simulink model "ODE1_zad1"  (Simulink 6.3)
settings: Solver=ode45  StartTime=0.0  StopTime=1  RelTol=1e-3
settings Model: LastModifiedBy=Ms1

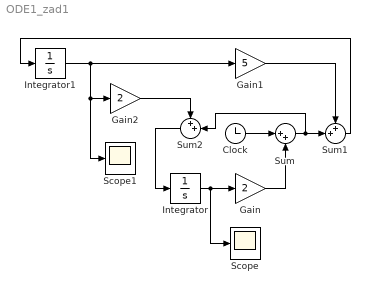
== system ODE1_zad1 ==
  Clock : Clock
      settings: Decimation=10
  Gain : Gain  Gain=2  SaturateOnIntegerOverflow=on
  Gain1 : Gain  Gain=5  SaturateOnIntegerOverflow=on
  Gain2 : Gain  Gain=2  SaturateOnIntegerOverflow=on
  Integrator : Integrator  InitialCondition=2
  Integrator1 : Integrator  InitialCondition=1
  Scope : Scope
  Scope1 : Scope
  Sum : Sum  Inputs=|++  SaturateOnIntegerOverflow=on  InputSameDT=on
  Sum1 : Sum  Inputs=++|  SaturateOnIntegerOverflow=on  InputSameDT=on
  Sum2 : Sum  Orientation=left  Inputs=++|  SaturateOnIntegerOverflow=on  InputSameDT=on
  wires:
  Clock/1 -> Sum/1
  Integrator/1 -> Gain/1, Scope/1
  Gain/1 -> Sum/2
  Integrator1/1 -> Gain1/1, Gain2/1, Scope1/1
  Sum/1 -> Sum1/2, Sum2/2
  Gain1/1 -> Sum1/1
  Sum1/1 -> Integrator1/1
  Gain2/1 -> Sum2/1
  Sum2/1 -> Integrator/1
